simulink model "Wiper_SystemModel"  (R2022b)
settings: Solver=VariableStepAuto  StartTime=0.0  StopTime=10.0  RelTol=1e-3
PreLoadFcn:
  | %Load Wiper Input & Output Bus
  | load('Wiper_InputOutput_Bus.mat');
settings Model: Creator=salman  LastModifiedBy=salman

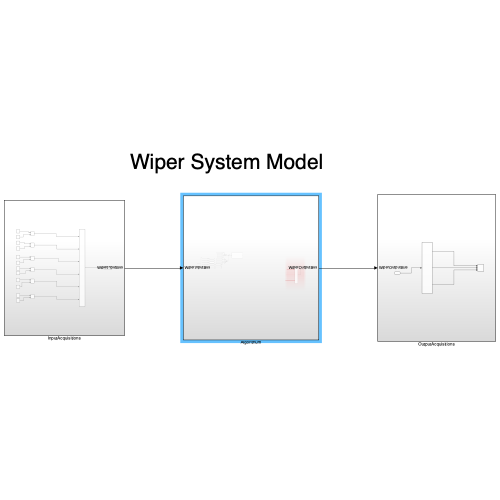
[thumbnail: Simulink's stored preview of the top-level diagram]
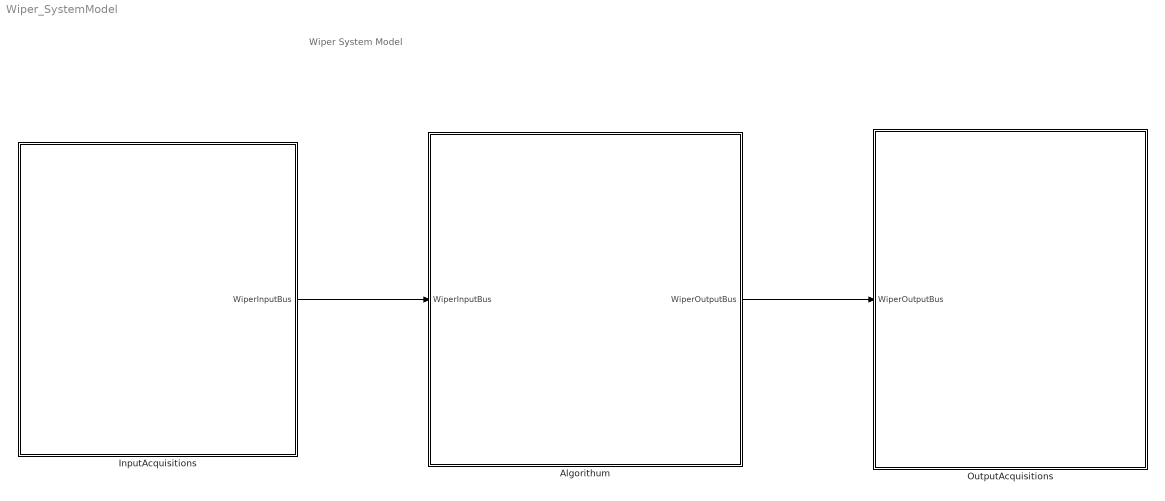
== system Wiper_SystemModel ==
  note: Wiper System Model
  Algorithum : Subsystem
  InputAcquisitions : Subsystem
  OutputAcquisitions : Subsystem
  wires:
  InputAcquisitions/1(WiperInputBus) -> Algorithum/1(WiperInputBus)
  Algorithum/1(WiperOutputBus) -> OutputAcquisitions/1(WiperOutputBus)

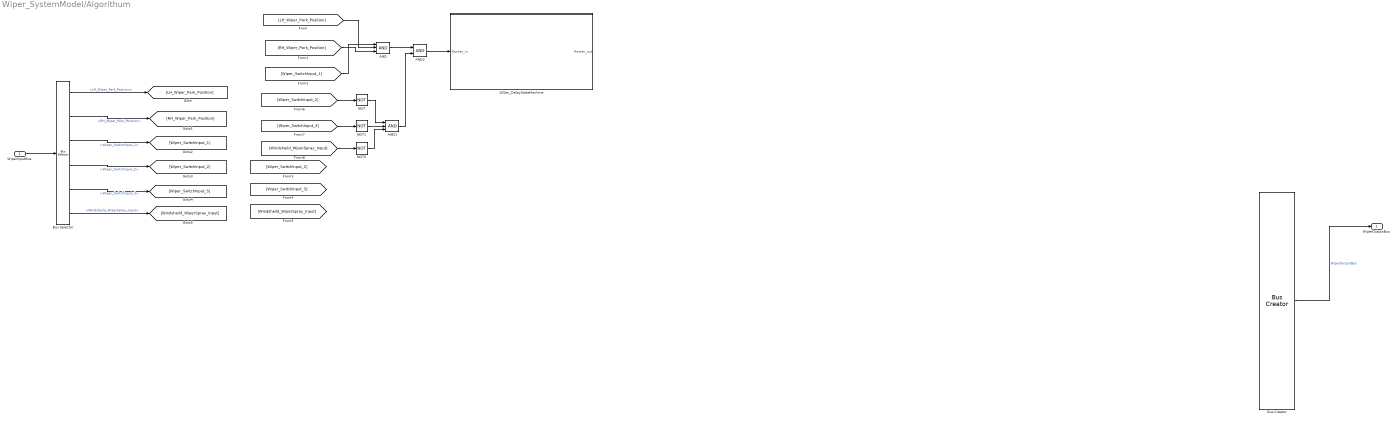
== system Wiper_SystemModel/Algorithum ==
  WiperInputBus : Inport  OutDataTypeStr=Bus: WiperInputBus
  10Sec_DelayStateMachine : Stateflow chart  TreatAsAtomicUnit=on  mask{delay=10}
      mask prompts: delay "Enter Delay Time"
  AND : Logic  Inputs=3  AllPortsSameDT=off  OutDataTypeStr=boolean
  AND1 : Logic  Inputs=3  AllPortsSameDT=off  OutDataTypeStr=boolean
  AND2 : Logic  AllPortsSameDT=off  OutDataTypeStr=boolean
  Bus Creator : BusCreator  Inputs=3  OutDataTypeStr=Bus: WiperOutputBus  NonVirtualBus=on
  Bus Selector : BusSelector  OutputSignals=LH_Wiper_Park_Position,RH_Wiper_Park_Position,Wiper_SwitchInput_1,Wiper_SwitchInput_2,Wiper_SwitchInput_3,Windsheild_WiperSpray_Input
  NOT : Logic  Operator=NOT  IconShape=distinctive  AllPortsSameDT=off  OutDataTypeStr=boolean
  NOT1 : Logic  Operator=NOT  IconShape=distinctive  AllPortsSameDT=off  OutDataTypeStr=boolean
  NOT2 : Logic  Operator=NOT  IconShape=distinctive  AllPortsSameDT=off  OutDataTypeStr=boolean
  WiperOutputBus : Outport  OutDataTypeStr=Bus: WiperOutputBus
  wires:
  WiperInputBus/1 -> Bus Selector/1
  Bus Selector/1 -> [LH_Wiper_Park_Position]  "<LH_Wiper_Park_Position>"
  Bus Selector/2 -> [RH_Wiper_Park_Position]  "<RH_Wiper_Park_Position>"
  Bus Selector/3 -> [Wiper_SwitchInput_1]  "<Wiper_SwitchInput_1>"
  Bus Selector/4 -> [Wiper_SwitchInput_2]  "<Wiper_SwitchInput_2>"
  Bus Selector/5 -> [Wiper_SwitchInput_3]  "<Wiper_SwitchInput_3>"
  Bus Selector/6 -> [Windsheild_WiperSpray_Input]  "<Windsheild_WiperSpray_Input>"
  ? -> Bus Creator/1  "LH_Wiper_Output"
  ? -> Bus Creator/2  "RH_Wiper_Output"
  ? -> Bus Creator/3  "WindsheildSpray_Output"
  Bus Creator/1 -> WiperOutputBus/1  "WiperOutputBus"
  AND/1 -> AND2/1
  [LH_Wiper_Park_Position] -> AND/2
  [RH_Wiper_Park_Position] -> AND/3
  [Wiper_SwitchInput_1] -> AND/1
  [Wiper_SwitchInput_2] -> NOT/1
  [Wiper_SwitchInput_3] -> NOT1/1
  [Windsheild_WiperSpray_Input] -> NOT2/1
  NOT/1 -> AND1/1
  NOT1/1 -> AND1/2
  NOT2/1 -> AND1/3
  AND1/1 -> AND2/2
  AND2/1 -> 10Sec_DelayStateMachine/1(flasher_in)

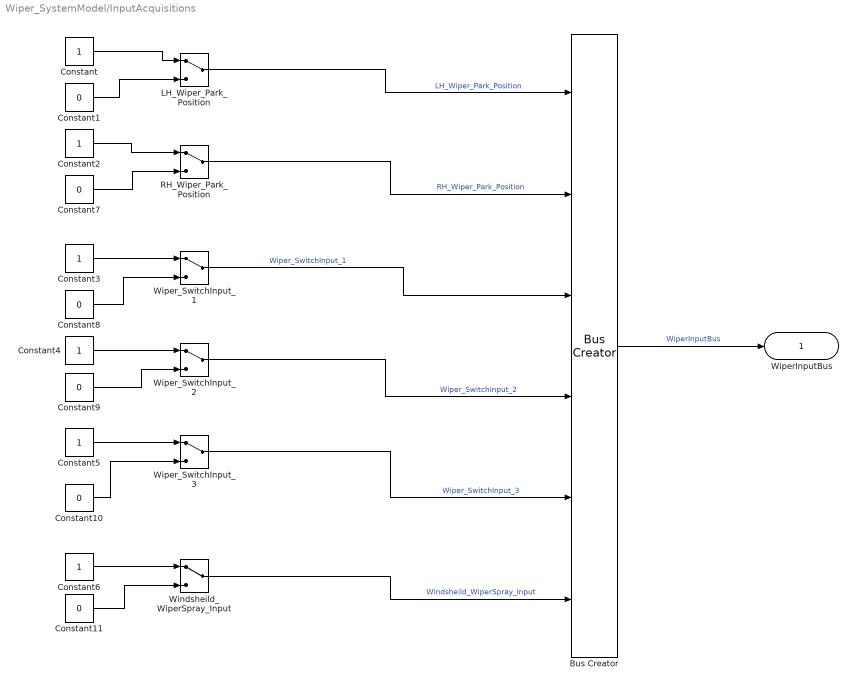
== system Wiper_SystemModel/InputAcquisitions ==
  Bus Creator : BusCreator  Inputs=6  OutDataTypeStr=Bus: WiperInputBus  NonVirtualBus=on
  Constant{,2..6} (6 alike) : Constant  OutDataTypeStr=boolean
  Constant{1,7..11} (6 alike) : Constant  Value=0  OutDataTypeStr=boolean
  LH_Wiper_Park_Position : ManualSwitch
  RH_Wiper_Park_Position : ManualSwitch
  Windsheild_WiperSpray_Input : ManualSwitch
  Wiper_SwitchInput_1 : ManualSwitch
  Wiper_SwitchInput_2 : ManualSwitch
  Wiper_SwitchInput_3 : ManualSwitch
  WiperInputBus : Outport  OutDataTypeStr=Bus: WiperInputBus
  wires:
  Constant/1 -> LH_Wiper_Park_Position/1
  Constant1/1 -> LH_Wiper_Park_Position/2
  Constant6/1 -> Windsheild_WiperSpray_Input/1
  Constant5/1 -> Wiper_SwitchInput_3/1
  Constant4/1 -> Wiper_SwitchInput_2/1
  Constant3/1 -> Wiper_SwitchInput_1/1
  Constant2/1 -> RH_Wiper_Park_Position/1
  Constant11/1 -> Windsheild_WiperSpray_Input/2
  Constant10/1 -> Wiper_SwitchInput_3/2
  Constant9/1 -> Wiper_SwitchInput_2/2
  Constant8/1 -> Wiper_SwitchInput_1/2
  Constant7/1 -> RH_Wiper_Park_Position/2
  LH_Wiper_Park_Position/1 -> Bus Creator/1  "LH_Wiper_Park_Position"
  RH_Wiper_Park_Position/1 -> Bus Creator/2  "RH_Wiper_Park_Position"
  Wiper_SwitchInput_1/1 -> Bus Creator/3  "Wiper_SwitchInput_1"
  Wiper_SwitchInput_2/1 -> Bus Creator/4  "Wiper_SwitchInput_2"
  Wiper_SwitchInput_3/1 -> Bus Creator/5  "Wiper_SwitchInput_3"
  Windsheild_WiperSpray_Input/1 -> Bus Creator/6  "Windsheild_WiperSpray_Input"
  Bus Creator/1 -> WiperInputBus/1  "WiperInputBus"

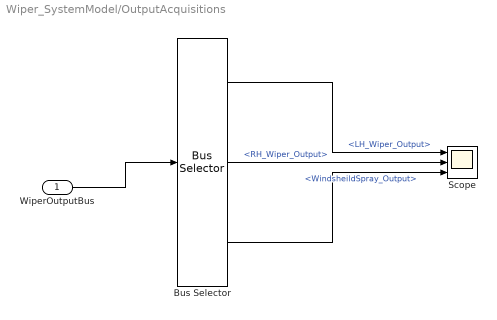
== system Wiper_SystemModel/OutputAcquisitions ==
  WiperOutputBus : Inport  OutDataTypeStr=Bus: WiperOutputBus
  Bus Selector : BusSelector  OutputSignals=LH_Wiper_Output,RH_Wiper_Output,WindsheildSpray_Output
  Scope : Scope  NumInputPorts=3
  wires:
  WiperOutputBus/1 -> Bus Selector/1
  Bus Selector/1 -> Scope/1  "<LH_Wiper_Output>"
  Bus Selector/2 -> Scope/2  "<RH_Wiper_Output>"
  Bus Selector/3 -> Scope/3  "<WindsheildSpray_Output>"

== stateflow chart Wiper_SystemModel/Algorithum/10Sec_DelayStateMachine ==
  state Idle
    entry:
    flasher_out = 0;
  state OFF
    entry:
    flasher_out=0;
  state ON
    entry:
    flasher_out = 1;
  (default) -> Idle
  Idle -> ON : [flasher_in==1]
  OFF -> Idle [order 2] : [flasher_in == 0]
  ON -> OFF : [after(delay,sec) || flasher_in == 0]
  OFF -> ON [order 1] : [after(delay,sec) && flasher_in ==1]
  data: flasher_in input; flasher_out output; delay parameter
